simulink model "solar"  (R2023b)
settings: Solver=VariableStepAuto  StartTime=0.0  StopTime=20  RelTol=1e-3
libraries: spsSeriesRLCBranchLib x8, spsIGBTDiodeLib x7, spsVoltageMeasurementLib x6, spsDiodeLib x5, spsRMSLib x3, spsCurrentMeasurementLib x2, simulink x1, spsPVArrayLib x1, sps_lib x1
settings Model: Creator=oiaon  LastModifiedBy=oiaon

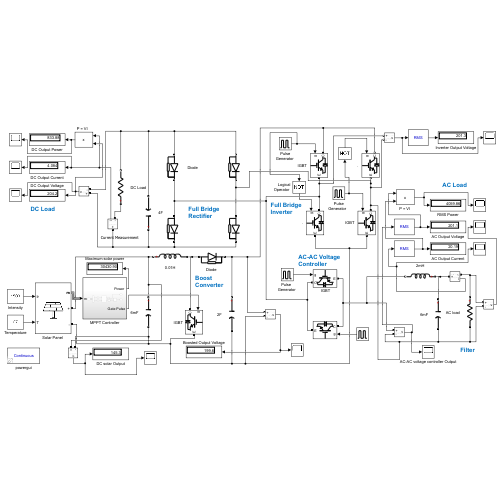
[thumbnail: Simulink's stored preview of the top-level diagram]
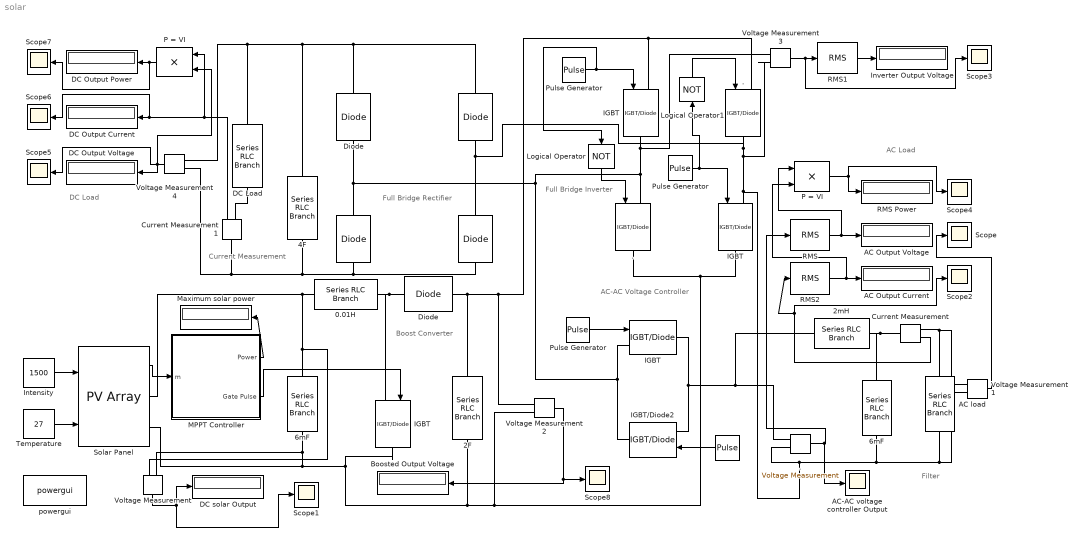
== system solar ==
  note: Current Measurement
  note: Full Bridge Inverter
  note: Full Bridge Rectifier
  note: AC-AC Voltage
      | Controller
  note: Filter
  note: Boost
      | Converter
  note: DC Load
  note: AC Load
  " " : spsDiodeLib/Diode  Ron=0.001  Lon=0  Vf=0.8  IC=0  UseSnubber=0  Rs=500  Cs=250e-9  Measurements=off
  "  " : spsDiodeLib/Diode  Ron=0.001  Lon=0  Vf=0.8  IC=0  UseSnubber=0  Rs=500  Cs=250e-9  Measurements=off
  "    " : spsDiodeLib/Diode  Ron=0.001  Lon=0  Vf=0.8  IC=0  UseSnubber=0  Rs=500  Cs=250e-9  Measurements=off
  "     " : DiscretePulseGenerator  PulseType=Time based  Period=1/60  PulseWidth=50  PhaseDelay=(1/60)*(180+1)/360
  "  Diode" : spsDiodeLib/Diode  Ron=0.001  Lon=0  Vf=0.8  IC=0  UseSnubber=0  Rs=500  Cs=250e-9  Measurements=off
  " . " : spsIGBTDiodeLib/IGBT//Diode  Ron=1e-3  Rs=1e5  Cs=inf  Measurements=off
  " 6mF" : spsSeriesRLCBranchLib/Series RLC Branch  LConnTagsString=__new0  RConnTagsString=__new0  BranchType=C  Resistance=0.0001  Inductance=1e-3  SetiL0=off  InitialCurrent=0  Capacitance=0.006  Setx0=off  InitialVoltage=0  Measurements=None
  " IGBT" : spsIGBTDiodeLib/IGBT//Diode  Ron=1e-3  Rs=1e5  Cs=inf  Measurements=off
  " IGBT " : spsIGBTDiodeLib/IGBT//Diode  Ron=1e-3  Rs=1e5  Cs=inf  Measurements=off
  . : spsVoltageMeasurementLib/Voltage Measurement  PhasorSimulation=off  OutputType=Complex  PSBequivalent=0
  ". " : spsIGBTDiodeLib/IGBT//Diode  Ron=1e-3  Rs=1e5  Cs=inf  Measurements=off
  0.01H : spsSeriesRLCBranchLib/Series RLC Branch  LConnTagsString=__new0  RConnTagsString=__new0  BranchType=L  Resistance=1  Inductance=0.1  SetiL0=off  InitialCurrent=0  Capacitance=1e-6  Setx0=off  InitialVoltage=0  Measurements=None
  2F : spsSeriesRLCBranchLib/Series RLC Branch  LConnTagsString=__new0  RConnTagsString=__new0  BranchType=C  Resistance=1  Inductance=0.003  SetiL0=off  InitialCurrent=0  Capacitance=2  Setx0=off  InitialVoltage=0  Measurements=None
  2mH : spsSeriesRLCBranchLib/Series RLC Branch  LConnTagsString=__new0  RConnTagsString=__new0  BranchType=L  Resistance=0.0001  Inductance=0.002  SetiL0=off  InitialCurrent=0  Capacitance=0.006  Setx0=off  InitialVoltage=0  Measurements=None
  4F : spsSeriesRLCBranchLib/Series RLC Branch  LConnTagsString=__new0  RConnTagsString=__new0  BranchType=C  Resistance=1  Inductance=1e-3  SetiL0=off  InitialCurrent=0  Capacitance=4  Setx0=off  InitialVoltage=0  Measurements=None
  6mF : spsSeriesRLCBranchLib/Series RLC Branch  LConnTagsString=__new0  RConnTagsString=__new0  BranchType=C  Resistance=0.0001  Inductance=1e-3  SetiL0=off  InitialCurrent=0  Capacitance=0.006  Setx0=off  InitialVoltage=0  Measurements=None
  AC Output Current : Display
  AC Output Voltage : Display
  AC load : spsSeriesRLCBranchLib/Series RLC Branch  LConnTagsString=__new0  RConnTagsString=__new0  BranchType=R  Resistance=50  Inductance=1e-3  SetiL0=off  InitialCurrent=0  Capacitance=0.006  Setx0=off  InitialVoltage=0  Measurements=None
  AC-AC voltage controller Output : Scope
  Boosted Output Voltage : Display
  Current Measurement : spsCurrentMeasurementLib/Current Measurement  PhasorSimulation=off  OutputType=Complex  PSBequivalent=0
  Current Measurement1 : spsCurrentMeasurementLib/Current Measurement  PhasorSimulation=off  OutputType=Complex  PSBequivalent=0
  DC Load : spsSeriesRLCBranchLib/Series RLC Branch  LConnTagsString=__new0  RConnTagsString=__new0  BranchType=R  Resistance=50  Inductance=1e-3  SetiL0=off  InitialCurrent=0  Capacitance=1e-6  Setx0=off  InitialVoltage=0  Measurements=None
  DC Output Current : Display
  DC Output Power : Display
      settings: Format=bank
  DC Output Voltage : Display
  DC solar Output : Display
  "Diode " : spsDiodeLib/Diode  Ron=0.001  Lon=0  Vf=0.8  IC=0  UseSnubber=0  Rs=500  Cs=250e-9  Measurements=off
  IGBT : spsIGBTDiodeLib/IGBT//Diode  Ron=1e-3  Rs=1e5  Cs=inf  Measurements=off
  "IGBT " : spsIGBTDiodeLib/IGBT//Diode  Ron=1e-3  Rs=1e5  Cs=inf  Measurements=off
  IGBT/Diode2 : spsIGBTDiodeLib/IGBT//Diode  Ron=1e-3  Rs=1e5  Cs=inf  Measurements=off
  Intensity : Constant  Value=1500
  Inverter Output Voltage : Display
  "Logical Operator " : Logic  Operator=NOT  AllPortsSameDT=off  OutDataTypeStr=boolean
  Logical Operator1 : Logic  Operator=NOT  AllPortsSameDT=off  OutDataTypeStr=boolean
  MPPT Controller : Subsystem
  Maximum solar power : Display
      settings: Format=bank
  "P = VI " : Product
  "P = VI   " : Product
  "Pulse Generator " : DiscretePulseGenerator  PulseType=Time based  Period=0.02  PulseWidth=50
  "Pulse Generator   " : DiscretePulseGenerator  PulseType=Time based  Period=0.02  PulseWidth=50
  "Pulse Generator " : DiscretePulseGenerator  PulseType=Time based  Period=1/60  PulseWidth=50  PhaseDelay=(1/60)*(1/360)
  RMS : spsRMSLib/RMS  TrueRMS=on  Freq=60  RMSInit=120  Ts=0
  RMS Power : Display
      settings: Format=bank
  RMS1 : spsRMSLib/RMS  TrueRMS=on  Freq=60  RMSInit=120  Ts=0
  RMS2 : spsRMSLib/RMS  TrueRMS=on  Freq=60  RMSInit=120  Ts=0
  Scope{,1..8} (9 alike) : Scope
  "Solar Panel " : spsPVArrayLib/PV Array  Npar=20  Nser=5  PlotType=array @ 1000 W/m2 & specified temperatures  S_vec="[ 1000  500  100 ]"  Temp_C_vec="[ 45 25  ]"  ModuleName=User-defined  PlotWhenSelected=off  Pm=213.15  Ncell=60  Voc=36.3  Isc=7.84  Vm=29  Im=7.35  beta_Voc_pc=-0.36099  alpha_Isc_pc=0.102  beta_Voc=-0.13104  alpha_Isc=0.0079968  IL=7.8654  I0=2.9273e-10  nI=0.98119  Rsh=313.0553  Rs=0.39381  RobustModel=off  RobustCellTemperature=313.3991  BAL=on  Tc=1e-6  Tfilter=5e-5
  Temperature : Constant  Value=27
  Voltage Measurement{,1..4} (5 alike) : spsVoltageMeasurementLib/Voltage Measurement  PhasorSimulation=off  OutputType=Complex  PSBequivalent=0
  powergui : sps_lib/powergui  Priority=1  SimulationMode=Continuous  SampleTime=50e-6  frequency=60  Iterations=50  frequencyindice=0  Pbase=100e6  ErrMax=1e-4  UnitsV=kV  UnitsW=MW  buscounter=0  FunctionMessages=off  echomessages=off  EnableUseOfTLC=off  CurrentSourceSwitches=off  DisableSnubberDevices=off  DisableRonSwitches=off  DisableVfSwitches=off  DisplayEquations=off  AutomaticDiscreteSolvers=off  SolverType=Tustin/Backward Euler (TBE)  Interpol=off  ExternalGateDelay=off  methode=off  Ts=100  x0status=blocks  SPID=on  SwTol=0  HookPort=off  NonlinearTolerance=1e-4  nMaxIteration=100  ContinueOnMaxIteration=off  RestoreLinks=warning  ResistiveCurrentMeasurement=off  Frange=[0:2:500]  Ylog=off  Xlog=on  ShowGrid=off  save=off  variable=ZData  structure=0  ZoomFFT=off  StartTime=0.0  cycles=1  DisplayStyle=1  fundamental=60  FreqAxis=off  MaxFrequency=1000  frequencyindicesteady=1  RmsSteady=1  display=off
  wires:
  Intensity/1 -> "Solar Panel "/1
  Temperature/1 -> "Solar Panel "/2
  Voltage Measurement/1 -> DC solar Output/1, Scope1/1
  ./1 -> AC-AC voltage controller Output/1, RMS/1
  Logical Operator1/1 -> ". "/1
  "Logical Operator "/1 -> " . "/1
  "Pulse Generator "/1 -> "Logical Operator "/1, " IGBT "/1
  "Pulse Generator   "/1 -> "IGBT "/1, Logical Operator1/1
  "Pulse Generator "/1 -> " IGBT"/1
  "     "/1 -> IGBT/Diode2/1
  RMS/1 -> "P = VI "/1, AC Output Voltage/1
  Voltage Measurement3/1 -> Scope3/1, RMS1/1
  RMS1/1 -> Inverter Output Voltage/1
  Voltage Measurement4/1 -> "P = VI   "/2, Scope5/1, DC Output Voltage/1
  Voltage Measurement1/1 -> Scope/1
  "Solar Panel "/1 -> MPPT Controller/1(m)
  MPPT Controller/2(Gate Pulse) -> IGBT/1
  MPPT Controller/1("Power ") -> Maximum solar power/1
  Current Measurement/1 -> RMS2/1, Scope2/1
  RMS2/1 -> "P = VI "/2, AC Output Current/1
  "P = VI "/1 -> RMS Power/1, Scope4/1
  Current Measurement1/1 -> "P = VI   "/1, Scope6/1, DC Output Current/1
  "P = VI   "/1 -> Scope7/1, DC Output Power/1
  Voltage Measurement2/1 -> Scope8/1, Boosted Output Voltage/1
  connections:
  0.01H/LConn1 -- Voltage Measurement/LConn1 -- 6mF/LConn1 -- "Solar Panel "/RConn1
  "Diode "/LConn1 -- IGBT/LConn1 -- 0.01H/RConn1
  " IGBT "/RConn1 -- Voltage Measurement3/LConn1 -- " . "/LConn1 -- "  Diode"/RConn1 -- " "/LConn1 -- IGBT/Diode2/RConn1 -- " IGBT"/LConn1
  "Diode "/RConn1 -- 2F/LConn1 -- Voltage Measurement2/LConn1 -- ". "/LConn1 -- " IGBT "/LConn1
  2mH/LConn1 -- Current Measurement/LConn1 -- " 6mF"/LConn1
  " IGBT"/RConn1 -- 2mH/RConn1 -- ./LConn1 -- IGBT/Diode2/LConn1
  Voltage Measurement4/LConn1 -- Current Measurement1/LConn1 -- 4F/LConn1 -- "    "/RConn1 -- " "/RConn1
  "  Diode"/LConn1 -- 4F/RConn1 -- DC Load/RConn1 -- Voltage Measurement4/LConn2 -- "  "/LConn1
  DC Load/LConn1 -- Current Measurement1/RConn1
  Current Measurement/RConn1 -- AC load/LConn1 -- Voltage Measurement1/LConn1
  " . "/RConn1 -- Voltage Measurement2/LConn2 -- 2F/RConn1 -- IGBT/RConn1 -- Voltage Measurement/LConn2 -- 6mF/RConn1 -- "Solar Panel "/RConn2 -- "IGBT "/RConn1
  "IGBT "/LConn1 -- "    "/LConn1 -- "  "/RConn1 -- ". "/RConn1 -- Voltage Measurement3/LConn2 -- ./LConn2 -- " 6mF"/RConn1 -- Voltage Measurement1/LConn2 -- AC load/RConn1

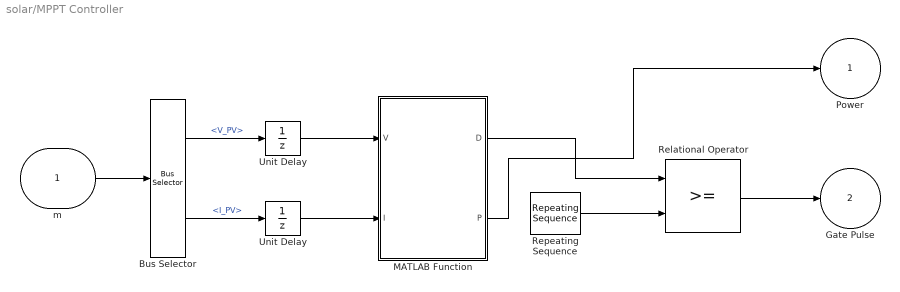
== system solar/MPPT Controller ==
  m : Inport
  "Bus Selector  " : BusSelector  OutputSignals=V_PV,I_PV
  "MATLAB Function " : MATLAB Function  TreatAsAtomicUnit=on
  "Relational Operator " : RelationalOperator  OutDataTypeStr=boolean  RndMeth=Simplest  InputSameDT=off
  "Repeating Sequence " : simulink/Sources/Repeating Sequence  rep_seq_t=[0 0.0002]  rep_seq_y=[0 1]
  "Unit Delay " : UnitDelay  SampleTime=1e-4  HasFrameUpgradeWarning=on
  "Unit Delay  " : UnitDelay  SampleTime=1e-4  HasFrameUpgradeWarning=on
  "Power " : Outport
  Gate Pulse : Outport  Port=2
  wires:
  m/1 -> "Bus Selector  "/1
  "Unit Delay "/1 -> "MATLAB Function "/1(V)
  "Relational Operator "/1 -> Gate Pulse/1
  "MATLAB Function "/1(D) -> "Relational Operator "/1
  "Unit Delay  "/1 -> "MATLAB Function "/2(I)
  "Bus Selector  "/1 -> "Unit Delay "/1  "<V_PV>"
  "Bus Selector  "/2 -> "Unit Delay  "/1  "<I_PV>"
  "MATLAB Function "/2(P) -> "Power "/1
  "Repeating Sequence "/1 -> "Relational Operator "/2

== matlab function solar/MPPT Controller/MATLAB Function  ==
  data: V input; D output; I input; P output
function [D, P] = DutyRatio(V, I)

Dmax = 0.95;
Dmin = 0.05;
deltaD = 0.001;

persistent Vold Pold Dold

if isempty(Vold)
    Vold = V;
    Pold = V*I;
    Dold = 0.5;
end

P = V * I;          % Power output

dV = V - Vold;
dP = P - Pold;

if dP > 0
    if dV > 0
        D = Dold - deltaD;
    else
        D = Dold + deltaD;
    end
elseif dP < 0
    if dV > 0
        D = Dold + deltaD;
    else
        D = Dold - deltaD;
    end
else
    D = Dold;
end

D = max(min(D, Dmax), Dmin);

Dold = D;
Vold = V;
Pold = P;

end
